simulink library "INP_IMU_Prep_EB"  (R2023b)
settings: Solver=VariableStepAuto  StartTime=0.0  StopTime=10.0  RelTol=1e-3
undefined symbols (not defined in the file): INP_IMU_p_AVehLgtOfs_mps2, INP_IMU_p_AVehLgtSca_na
libraries: eeGeneralControl x1
settings Model: Creator=blatak  LastModifiedBy=blatak

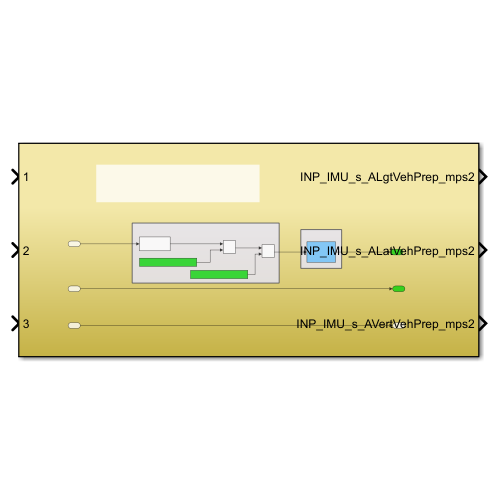
[thumbnail: Simulink's stored preview of the top-level diagram]
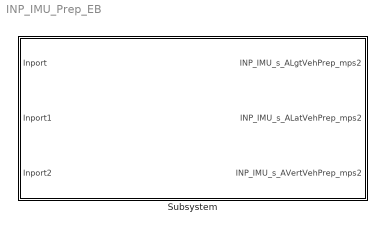
== system INP_IMU_Prep_EB ==
  Subsystem : Subsystem

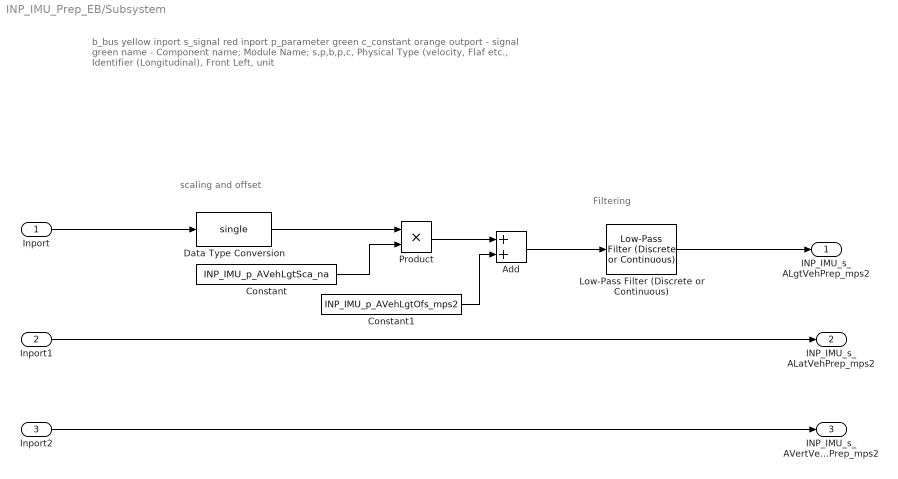
== system INP_IMU_Prep_EB/Subsystem ==
  note: scaling and offset
  note: b_bus yellow inport
      | s_signal red inport
      | p_parameter green
      | c_constant orange
      | outport - signal green
      | name - Component name; Module Name; s,p,b,p,c, Physical Type (velocity, Flaf etc., Identifier (Longitudinal), Front Left, unit
  note: Filtering
  Inport : Inport
  Inport1 : Inport  Port=2
  Inport2 : Inport  Port=3
  Add : Sum
  Constant : Constant  Value=INP_IMU_p_AVehLgtSca_na
  Constant1 : Constant  Value=INP_IMU_p_AVehLgtOfs_mps2
  Data Type Conversion : DataTypeConversion  OutDataTypeStr=single  SaturateOnIntegerOverflow=off  RndMeth=Floor
  Low-Pass Filter (Discrete or Continuous) : eeGeneralControl/Low-Pass Filter (Discrete or Continuous)  K=1  T=1  B=inf  A=-inf  init_option=Inherited from block input  x0=0  Ts=-1
  Product : Product
  INP_IMU_s_ALgtVehPrep_mps2 : Outport
  INP_IMU_s_ALatVehPrep_mps2 : Outport  Port=2
  INP_IMU_s_AVertVehPrep_mps2 : Outport  Port=3
  wires:
  Inport1/1 -> INP_IMU_s_ALatVehPrep_mps2/1
  Product/1 -> Add/1
  Data Type Conversion/1 -> Product/1
  Constant1/1 -> Add/2
  Constant/1 -> Product/2
  Inport/1 -> Data Type Conversion/1
  Low-Pass Filter (Discrete or Continuous)/1 -> INP_IMU_s_ALgtVehPrep_mps2/1
  Add/1 -> Low-Pass Filter (Discrete or Continuous)/1
  Inport2/1 -> INP_IMU_s_AVertVehPrep_mps2/1
